simulink model "example_simulink_send_receive"  (R2015b)
settings: Solver=FixedStepAuto  StartTime=0.0  StopTime=inf  FixedStep=1/75  RelTol=1e-3
undefined symbols (not defined in the file or in its folder): CR, LF, serial
libraries: instrumentlib x3, etargetslib x1, aerolibanimutils x1
settings Model: Creator=marcell  LastModifiedBy=marcell

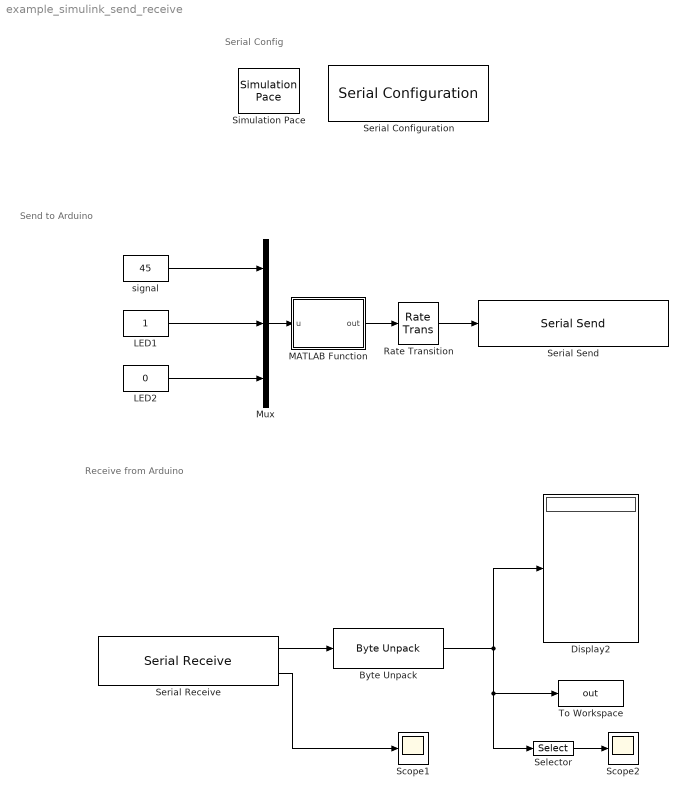
== system example_simulink_send_receive ==
  note: Send to Arduino
  note: Serial Config
  note: Receive from Arduino
  Byte Unpack : etargetslib/Byte Unpack  dimensions={[3]}  datatypes={'single'}  byteAlign=1
  Display2 : Display
  LED1 : Constant  OutDataTypeStr=single
  LED2 : Constant  Value=0  OutDataTypeStr=single
  MATLAB Function : MATLAB Function  TreatAsAtomicUnit=on
  Mux : Mux  Inputs=3
  Rate Transition : RateTransition  OutPortSampleTime=1/75
  Scope1 : Scope
  Scope2 : Scope
  Selector : Selector  InputPortWidth=3  IndexOptions=Index vector (dialog)  Indices=2  OutputSizes=1
  Serial Configuration : instrumentlib/Serial Configuration  Priority=-200000  ComPortMenu=<Please select a port...>  ComPort=/dev/tty.usbmodem1421  ObjConstructor=serial('/dev/tty.usbmodem1421');  BaudRate=115200  DataBits=8  Parity=none  StopBits=1  FlowControl=none  Timeout=10  ByteOrder=LittleEndian
  Serial Receive : instrumentlib/Serial Receive  ComPortMenu=<Please select a port...>  ComPort=/dev/tty.usbmodem1421  ObjConstructor=serial('/dev/tty.usbmodem1421');  Header=aaaaaaaa  Terminator=CR/LF ('\r\n')  DataSize="[1  12]"  DataType=uint8  EnableBlockingMode=off  ActionDataUnavailable=Output last received value  CustomValue=0  SampleTime=1/75
  Serial Send : instrumentlib/Serial Send  ComPortMenu=<Please select a port...>  ComPort=/dev/tty.usbmodem1421  ObjConstructor=serial('/dev/tty.usbmodem1421');  Header=bbbb  Terminator=CR/LF ('\r\n')  EnableBlockingMode=on
  Simulation Pace : aerolibanimutils/Simulation Pace  SimulationPace=1  SleepMode=MATLAB Thread  OutputPaceError=off  SampleTime=1/75
  To Workspace : ToWorkspace  VariableName=out  SaveFormat=Structure With Time  SampleTime=-1
  signal : Constant  Value=45  OutDataTypeStr=single
  wires:
  Byte Unpack/1 -> Selector/1, To Workspace/1, Display2/1
  Serial Receive/2 -> Scope1/1
  Rate Transition/1 -> Serial Send/1
  Serial Receive/1 -> Byte Unpack/1
  MATLAB Function/1(out) -> Rate Transition/1
  LED1/1 -> Mux/2
  signal/1 -> Mux/1
  Mux/1 -> MATLAB Function/1(u)
  LED2/1 -> Mux/3
  Selector/1 -> Scope2/1

== matlab function example_simulink_send_receive/MATLAB Function ==
  data: u input; out output
function out = fcn(u)

%#codegen
u_single = single(u);
u_byte = typecast(u_single,'uint8');
len_single = uint8(numel(u_single));
len_byte = uint8(numel(u_byte));
y = uint8(zeros((len_single*4)+1,1));
y(1) = len_byte;
for i = 1:len_byte
   y(i+1) = u_byte(i) ;
end
out = y;
